simulink model "lab_1_2_diag"  (R2023b)
settings: Solver=FixedStepAuto  StartTime=0.0  StopTime=10.0  FixedStep=0.0001  RelTol=1e-3
undefined symbols (not defined in the file): beta_1, beta_2, beta_3, lam_1, lam_2, lam_3
settings Model: Creator=nsukh  LastModifiedBy=nsukh

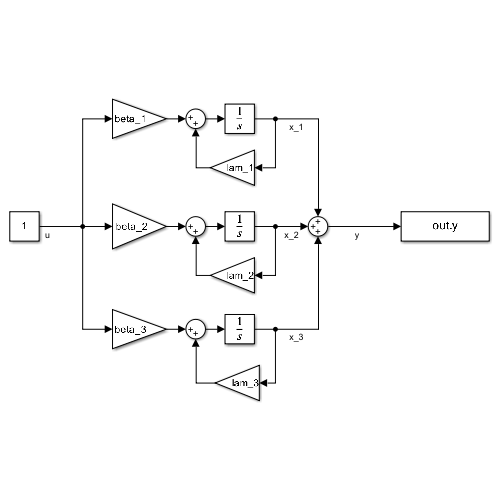
[thumbnail: Simulink's stored preview of the top-level diagram]
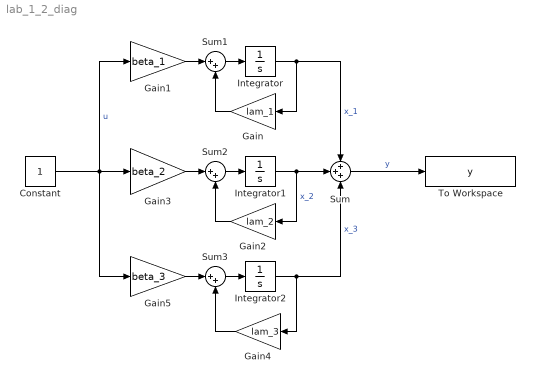
== system lab_1_2_diag ==
  Constant : Constant  SampleTime=-1
  Gain : Gain  Gain=lam_1
  Gain1 : Gain  Gain=beta_1
  Gain2 : Gain  Gain=lam_2
  Gain3 : Gain  Gain=beta_2
  Gain4 : Gain  Gain=lam_3
  Gain5 : Gain  Gain=beta_3
  Integrator : Integrator
  Integrator1 : Integrator
  Integrator2 : Integrator
  Sum : Sum  Inputs=+++
  Sum1 : Sum  Inputs=|++
  Sum2 : Sum  Inputs=|++
  Sum3 : Sum  Inputs=|++
  To Workspace : ToWorkspace  VariableName=y  SaveFormat=Timeseries  SampleTime=-1
  wires:
  Sum/1 -> To Workspace/1  "y"
  Integrator/1 -> Sum/1, Gain/1  "x_1"
  Gain1/1 -> Sum1/1
  Sum1/1 -> Integrator/1
  Gain/1 -> Sum1/2
  Gain2/1 -> Sum2/2
  Integrator1/1 -> Sum/2, Gain2/1  "x_2"
  Sum2/1 -> Integrator1/1
  Gain3/1 -> Sum2/1
  Gain4/1 -> Sum3/2
  Integrator2/1 -> Sum/3, Gain4/1  "x_3"
  Sum3/1 -> Integrator2/1
  Gain5/1 -> Sum3/1
  Constant/1 -> Gain5/1, Gain1/1, Gain3/1  "u"
